simulink model "FGC_Test_ROS"  (R2023a)
settings: Solver=ode3  StartTime=0.0  StopTime=inf  FixedStep=0.05  RelTol=1e-3
libraries: robotlib x4
settings Model: Creator=gptp  LastModifiedBy=gptp
settings OptimizationCC: EnhancedBackFolding=on  PassReuseOutputArgsAs=Individual arguments  ZeroExternalMemoryAtStartup=off  ZeroInternalMemoryAtStartup=off  MaxStackSize=64  OptimizeBlockOrder=speed  DifferentSizesBufferReuse=on  OptimizationCustomize=off  EfficientTunableParamExpr=on
settings DebuggingCC: ParameterTunabilityLossMsg=error
settings HardwareCC: ProdBitPerLong=64  ProdLargestAtomicInteger=LongLong  ProdLargestAtomicFloat=Double  ProdLongLongMode=on  ProdHWDeviceType=ARM Compatible->ARM 64-bit (LP64)
settings SFSimCC: MATLABDynamicMemAlloc=off
settings RTWCC: Description=Embedded Coder  SystemTargetFile=ert.tlc  HardwareBoard=Robot Operating System (ROS)  TLCOptions="-aInlineSetEventsForThisBaseRateFcn=TLC_FALSE -aSuppressMultiTaskScheduler=TLC_FALSE  -aRateBasedStepFcn=0"  GenCodeOnly=on  TemplateMakefile=ert_default_tmf  Toolchain=Catkin  TargetLang=C++
settings CodeAppCC: ForceParamTrailComments=on  IgnoreCustomStorageClasses=off  OperatorAnnotations=on  SimulinkDataObjDesc=on  SFDataObjDesc=on  InsertBlockDesc=on
settings ERTTargetCC: SupportVariableSizeSignals=on

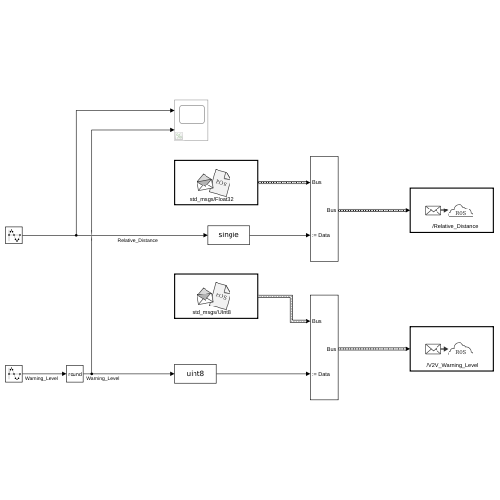
[thumbnail: Simulink's stored preview of the top-level diagram]
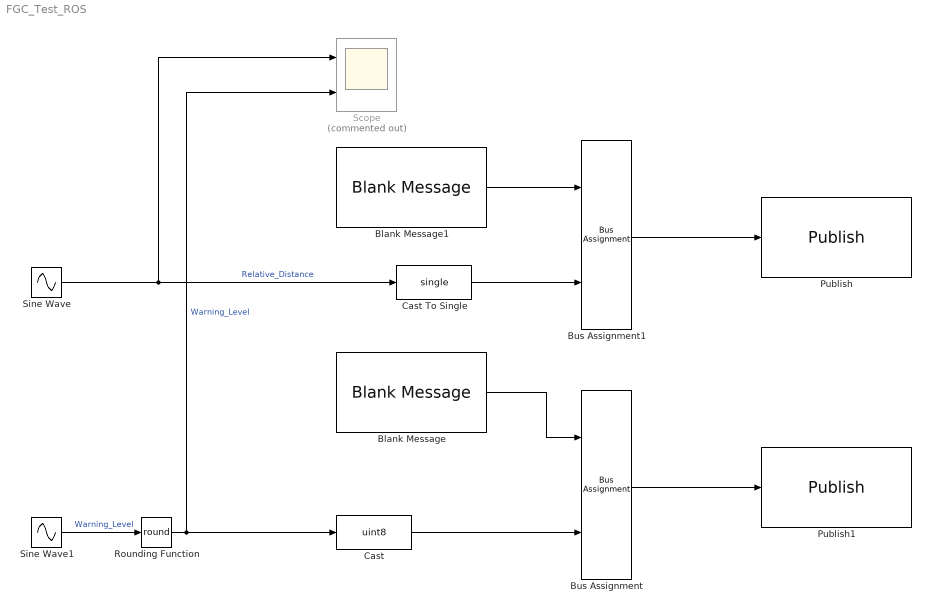
== system FGC_Test_ROS ==
  Blank Message : robotlib/Blank Message  messageClass=Message  entityType=std_msgs/UInt8  messageType=std_msgs/UInt8  SampleTime=inf  legacyBusStruct=off
  Blank Message1 : robotlib/Blank Message  messageClass=Message  entityType=std_msgs/Float32  messageType=std_msgs/Float32  SampleTime=inf  legacyBusStruct=off
  Bus Assignment : BusAssignment  AssignedSignals=Data
  Bus Assignment1 : BusAssignment  AssignedSignals=Data
  Cast : DataTypeConversion  OutDataTypeStr=uint8  SaturateOnIntegerOverflow=off  RndMeth=Floor
  Cast To Single : DataTypeConversion  OutDataTypeStr=single  SaturateOnIntegerOverflow=off  RndMeth=Floor
  Publish : robotlib/Publish  topicSource=Specify your own  topic=/Relative_Distance  messageType=std_msgs/Float32  legacyBusStruct=off  messageQueueLength=1
  Publish1 : robotlib/Publish  topicSource=Specify your own  topic=/V2V_Warning_Level  messageType=std_msgs/UInt8  legacyBusStruct=off  messageQueueLength=1
  Rounding Function : Rounding  Operator=round
  Scope : Scope  Commented=on  NumInputPorts=2
  Sine Wave : Sin  SineType=Sample based  Amplitude=50  Bias=50  Samples=100  SampleTime=0.1
  Sine Wave1 : Sin  SineType=Sample based  Amplitude=5  Bias=5  Samples=50  SampleTime=0.1
  wires:
  Blank Message/1 -> Bus Assignment/1
  Bus Assignment/1 -> Publish1/1
  Bus Assignment1/1 -> Publish/1
  Blank Message1/1 -> Bus Assignment1/1
  Sine Wave/1 -> Scope/1, Cast To Single/1  "Relative_Distance"
  Sine Wave1/1 -> Rounding Function/1  "Warning_Level"
  Rounding Function/1 -> Scope/2, Cast/1  "Warning_Level"
  Cast/1 -> Bus Assignment/2
  Cast To Single/1 -> Bus Assignment1/2
